simulink model "Hybrid_P2_Parallel"  (R2017b)
settings: Solver=FixedStepAuto  StartTime=0.0  StopTime=length(Speed)  FixedStep=0.01  MaxStep=0.01  RelTol=1e-3  EnableMultiTasking=on
PostLoadFcn:
  | , if any(exist('dsrtsu_mdlpostloadfcn', 'file') == [2, 3, 6]), try dsrtsu_mdlpostloadfcn('Execute', bdroot); catch fprintf('Error in PostLoadFcn (dsrtsu_mdlpostloadfcn) for model "%s":\n %s\n', bdroot, lasterr); end, end,
undefined symbols (not defined in the file): APP1_OOR, APP2_OOR, APP_Mismatch, Brk_Flt, cal, clt, Clutch, Clutch2, ClutchEngag, eng, Engine, EngOverTemp, ENGTRQ_MSMCH_Degraded_CP, ENGTRQ_MSMCH_ErrCritical_CP, ENGTRQ_MSMCH_LimpHome_CP, EngTrqMismatch, ess, ESSOverTemp, gb, KeyPos_Flt, LossCAN, MCUOverTemp, mot, MotDirMismatch, MotOverTemp, MotTrqMismatch, mph2kph, PRNDL_Flt, RegenFault, time, tloop
libraries: simulink x100, EC2_libraries x7, powerlib_meascontrol x2, lib_Actuators x1, CalculationGallon x1, lib_Chassis x1, autolibcoupling x1, autolibsharedcoupling x1, lib_DCDC x1, lib_Differential x1, lib_EMachine_2017a x1, lib_HVESS x1
(part 5 of 7)

== system Hybrid_P2_Parallel/Controller/HSC/Camaro Fault Detection/Input Conversions/BMS_Conversions/Override  closeContactorsCmd ==
  note: Override Switch Subsystem
  note: This subsystem is used to override the model value of a signal to a constant value
  In1 : Inport
  Multiport Switch : MultiPortSwitch  DataPortOrder=Zero-based contiguous  Inputs=2  zeroidx=on
  Override Value : Constant  Value=0  OutDataTypeStr=double
  Signal Override Switch 0 = Use Model 1 = Use Constant : Constant  Value=0
  Out1 : Outport
  wires:
  Override Value/1 -> Multiport Switch/3
  Multiport Switch/1 -> Out1/1
  In1/1 -> Multiport Switch/2
  Signal Override Switch 0 = Use Model 1 = Use Constant/1 -> Multiport Switch/1

== system Hybrid_P2_Parallel/Controller/HSC/Camaro Fault Detection/Input Conversions/BMS_Conversions/Override  contactorsClsd ==
  note: Override Switch Subsystem
  note: This subsystem is used to override the model value of a signal to a constant value
  In1 : Inport
  Multiport Switch : MultiPortSwitch  DataPortOrder=Zero-based contiguous  Inputs=2  zeroidx=on
  Override Value : Constant  Value=0  OutDataTypeStr=double
  Signal Override Switch 0 = Use Model 1 = Use Constant : Constant  Value=0
  Out1 : Outport
  wires:
  Override Value/1 -> Multiport Switch/3
  Multiport Switch/1 -> Out1/1
  In1/1 -> Multiport Switch/2
  Signal Override Switch 0 = Use Model 1 = Use Constant/1 -> Multiport Switch/1

== system Hybrid_P2_Parallel/Controller/HSC/Camaro Fault Detection/Input Conversions/BMS_Conversions/Override  essCur_A ==
  note: This subsystem is used to override the model value of a signal to a constant value
  note: Override Switch Subsystem
  In1 : Inport
  Multiport Switch : MultiPortSwitch  DataPortOrder=Zero-based contiguous  Inputs=2  zeroidx=on
  Override Value : Constant  Value=0  OutDataTypeStr=double
  Signal Override Switch 0 = Use Model 1 = Use Constant : Constant  Value=0
  Out1 : Outport
  wires:
  Signal Override Switch 0 = Use Model 1 = Use Constant/1 -> Multiport Switch/1
  In1/1 -> Multiport Switch/2
  Multiport Switch/1 -> Out1/1
  Override Value/1 -> Multiport Switch/3

== system Hybrid_P2_Parallel/Controller/HSC/Camaro Fault Detection/Input Conversions/BMS_Conversions/Override  essSOC_0_1 ==
  note: Override Switch Subsystem
  note: This subsystem is used to override the model value of a signal to a constant value
  In1 : Inport
  Multiport Switch : MultiPortSwitch  DataPortOrder=Zero-based contiguous  Inputs=2  zeroidx=on
  Override Value : Constant  Value=0  OutDataTypeStr=double
  Signal Override Switch 0 = Use Model 1 = Use Constant : Constant  Value=0
  Out1 : Outport
  wires:
  Override Value/1 -> Multiport Switch/3
  Multiport Switch/1 -> Out1/1
  In1/1 -> Multiport Switch/2
  Signal Override Switch 0 = Use Model 1 = Use Constant/1 -> Multiport Switch/1

== system Hybrid_P2_Parallel/Controller/HSC/Camaro Fault Detection/Input Conversions/BMS_Conversions/Override  essTemp_C ==
  note: Override Switch Subsystem
  note: This subsystem is used to override the model value of a signal to a constant value
  In1 : Inport
  Multiport Switch : MultiPortSwitch  DataPortOrder=Zero-based contiguous  Inputs=2  zeroidx=on
  Override Value : Constant  Value=0  OutDataTypeStr=double
  Signal Override Switch 0 = Use Model 1 = Use Constant : Constant
  Out1 : Outport
  wires:
  Override Value/1 -> Multiport Switch/3
  Multiport Switch/1 -> Out1/1
  In1/1 -> Multiport Switch/2
  Signal Override Switch 0 = Use Model 1 = Use Constant/1 -> Multiport Switch/1

== system Hybrid_P2_Parallel/Controller/HSC/Camaro Fault Detection/Input Conversions/BMS_Conversions/Override  hvBattVolt_V ==
  note: Override Switch Subsystem
  note: This subsystem is used to override the model value of a signal to a constant value
  In1 : Inport
  Multiport Switch : MultiPortSwitch  DataPortOrder=Zero-based contiguous  Inputs=2  zeroidx=on
  Override Value : Constant  Value=0  OutDataTypeStr=double
  Signal Override Switch 0 = Use Model 1 = Use Constant : Constant  Value=0
  Out1 : Outport
  wires:
  Override Value/1 -> Multiport Switch/3
  Multiport Switch/1 -> Out1/1
  In1/1 -> Multiport Switch/2
  Signal Override Switch 0 = Use Model 1 = Use Constant/1 -> Multiport Switch/1

== system Hybrid_P2_Parallel/Controller/HSC/Camaro Fault Detection/Input Conversions/BMS_Conversions/Override  hvBusVolt_V ==
  note: This subsystem is used to override the model value of a signal to a constant value
  note: Override Switch Subsystem
  In1 : Inport
  Multiport Switch : MultiPortSwitch  DataPortOrder=Zero-based contiguous  Inputs=2  zeroidx=on
  Override Value : Constant  Value=0  OutDataTypeStr=double
  Signal Override Switch 0 = Use Model 1 = Use Constant : Constant  Value=0
  Out1 : Outport
  wires:
  Signal Override Switch 0 = Use Model 1 = Use Constant/1 -> Multiport Switch/1
  In1/1 -> Multiport Switch/2
  Multiport Switch/1 -> Out1/1
  Override Value/1 -> Multiport Switch/3

== system Hybrid_P2_Parallel/Controller/HSC/Camaro Fault Detection/Input Conversions/BMS_Conversions/Override  rollingAliveCnt [1_3] ==
  note: This subsystem is used to override the model value of a signal to a constant value
  note: Override Switch Subsystem
  In1 : Inport
  Multiport Switch : MultiPortSwitch  DataPortOrder=Zero-based contiguous  Inputs=2  zeroidx=on
  Override Value : Constant  Value=0  OutDataTypeStr=double
  Signal Override Switch 0 = Use Model 1 = Use Constant : Constant  Value=0
  Out1 : Outport
  wires:
  Signal Override Switch 0 = Use Model 1 = Use Constant/1 -> Multiport Switch/1
  In1/1 -> Multiport Switch/2
  Multiport Switch/1 -> Out1/1
  Override Value/1 -> Multiport Switch/3

== system Hybrid_P2_Parallel/Controller/HSC/Camaro Fault Detection/Input Conversions/BMS_Conversions/Override Fehler_HS_offen ==
  note: Override Switch Subsystem
  note: This subsystem is used to override the model value of a signal to a constant value
  In1 : Inport
  Multiport Switch : MultiPortSwitch  DataPortOrder=Zero-based contiguous  Inputs=2  zeroidx=on
  Override Value : Constant  Value=0  OutDataTypeStr=double
  Signal Override Switch 0 = Use Model 1 = Use Constant : Constant
  Out1 : Outport
  wires:
  Override Value/1 -> Multiport Switch/3
  Multiport Switch/1 -> Out1/1
  In1/1 -> Multiport Switch/2
  Signal Override Switch 0 = Use Model 1 = Use Constant/1 -> Multiport Switch/1

== system Hybrid_P2_Parallel/Controller/HSC/Camaro Fault Detection/Input Conversions/BMS_Conversions/Override Fehler_HS_verschweisst ==
  note: This subsystem is used to override the model value of a signal to a constant value
  note: Override Switch Subsystem
  In1 : Inport
  Multiport Switch : MultiPortSwitch  DataPortOrder=Zero-based contiguous  Inputs=2  zeroidx=on
  Override Value : Constant  Value=0  OutDataTypeStr=double
  Signal Override Switch 0 = Use Model 1 = Use Constant : Constant
  Out1 : Outport
  wires:
  Signal Override Switch 0 = Use Model 1 = Use Constant/1 -> Multiport Switch/1
  In1/1 -> Multiport Switch/2
  Multiport Switch/1 -> Out1/1
  Override Value/1 -> Multiport Switch/3

== system Hybrid_P2_Parallel/Controller/HSC/Camaro Fault Detection/Input Conversions/DriverInput_Conversions/Override  KeyPos [0_3] ==
  note: This subsystem is used to override the model value of a signal to a constant value
  note: Override Switch Subsystem
  In1 : Inport
  Multiport Switch : MultiPortSwitch  DataPortOrder=Zero-based contiguous  Inputs=2  zeroidx=on
  Override Value : Constant  Value=0  OutDataTypeStr=double
  Signal Override Switch 0 = Use Model 1 = Use Constant : Constant  Value=0
  Out1 : Outport
  wires:
  Signal Override Switch 0 = Use Model 1 = Use Constant/1 -> Multiport Switch/1
  In1/1 -> Multiport Switch/2
  Multiport Switch/1 -> Out1/1
  Override Value/1 -> Multiport Switch/3

== system Hybrid_P2_Parallel/Controller/HSC/Camaro Fault Detection/Input Conversions/DriverInput_Conversions/Override APP (%) ==
  note: This subsystem is used to override the model value of a signal to a constant value
  note: Override Switch Subsystem
  In1 : Inport
  Multiport Switch : MultiPortSwitch  DataPortOrder=Zero-based contiguous  Inputs=2  zeroidx=on
  Override Value : Constant  Value=0  OutDataTypeStr=double
  Signal Override Switch 0 = Use Model 1 = Use Constant : Constant  Value=0
  Out1 : Outport
  wires:
  Signal Override Switch 0 = Use Model 1 = Use Constant/1 -> Multiport Switch/1
  In1/1 -> Multiport Switch/2
  Multiport Switch/1 -> Out1/1
  Override Value/1 -> Multiport Switch/3

== system Hybrid_P2_Parallel/Controller/HSC/Camaro Fault Detection/Input Conversions/DriverInput_Conversions/Override APP (%)1 ==
  note: Override Switch Subsystem
  note: This subsystem is used to override the model value of a signal to a constant value
  In1 : Inport
  Multiport Switch : MultiPortSwitch  DataPortOrder=Zero-based contiguous  Inputs=2  zeroidx=on
  Override Value : Constant  Value=0  OutDataTypeStr=double
  Signal Override Switch 0 = Use Model 1 = Use Constant : Constant  Value=0
  Out1 : Outport
  wires:
  Override Value/1 -> Multiport Switch/3
  Multiport Switch/1 -> Out1/1
  In1/1 -> Multiport Switch/2
  Signal Override Switch 0 = Use Model 1 = Use Constant/1 -> Multiport Switch/1

== system Hybrid_P2_Parallel/Controller/HSC/Camaro Fault Detection/Input Conversions/DriverInput_Conversions/Override BPP (%) ==
  note: Override Switch Subsystem
  note: This subsystem is used to override the model value of a signal to a constant value
  In1 : Inport
  Multiport Switch : MultiPortSwitch  DataPortOrder=Zero-based contiguous  Inputs=2  zeroidx=on
  Override Value : Constant  Value=0  OutDataTypeStr=double
  Signal Override Switch 0 = Use Model 1 = Use Constant : Constant  Value=0
  Out1 : Outport
  wires:
  Override Value/1 -> Multiport Switch/3
  Multiport Switch/1 -> Out1/1
  In1/1 -> Multiport Switch/2
  Signal Override Switch 0 = Use Model 1 = Use Constant/1 -> Multiport Switch/1

== system Hybrid_P2_Parallel/Controller/HSC/Camaro Fault Detection/Input Conversions/DriverInput_Conversions/Override PRNDL ==
  note: This subsystem is used to override the model value of a signal to a constant value
  note: Override Switch Subsystem
  In1 : Inport
  Multiport Switch : MultiPortSwitch  DataPortOrder=Zero-based contiguous  Inputs=2  zeroidx=on
  Override Value : Constant  Value=0  OutDataTypeStr=double
  Signal Override Switch 0 = Use Model 1 = Use Constant : Constant  Value=0
  Out1 : Outport
  wires:
  Signal Override Switch 0 = Use Model 1 = Use Constant/1 -> Multiport Switch/1
  In1/1 -> Multiport Switch/2
  Multiport Switch/1 -> Out1/1
  Override Value/1 -> Multiport Switch/3

== system Hybrid_P2_Parallel/Controller/HSC/Camaro Fault Detection/Input Conversions/DriverInput_Conversions/Override Regen ==
  note: This subsystem is used to override the model value of a signal to a constant value
  note: Override Switch Subsystem
  In1 : Inport
  Multiport Switch : MultiPortSwitch  DataPortOrder=Zero-based contiguous  Inputs=2  zeroidx=on
  Override Value : Constant  Value=0  OutDataTypeStr=double
  Signal Override Switch 0 = Use Model 1 = Use Constant : Constant  Value=0
  Out1 : Outport
  wires:
  Signal Override Switch 0 = Use Model 1 = Use Constant/1 -> Multiport Switch/1
  In1/1 -> Multiport Switch/2
  Multiport Switch/1 -> Out1/1
  Override Value/1 -> Multiport Switch/3

== system Hybrid_P2_Parallel/Controller/HSC/Camaro Fault Detection/Input Conversions/DriverInput_Conversions/Override V [mph] ==
  note: Override Switch Subsystem
  note: This subsystem is used to override the model value of a signal to a constant value
  In1 : Inport
  Multiport Switch : MultiPortSwitch  DataPortOrder=Zero-based contiguous  Inputs=2  zeroidx=on
  Override Value : Constant  Value=0  OutDataTypeStr=double
  Signal Override Switch 0 = Use Model 1 = Use Constant : Constant  Value=0
  Out1 : Outport
  wires:
  Override Value/1 -> Multiport Switch/3
  Multiport Switch/1 -> Out1/1
  In1/1 -> Multiport Switch/2
  Signal Override Switch 0 = Use Model 1 = Use Constant/1 -> Multiport Switch/1

== system Hybrid_P2_Parallel/Controller/HSC/Camaro Fault Detection/Input Conversions/ECM_Conversions/Override  ECMTrqCmd_Nm ==
  note: Override Switch Subsystem
  note: This subsystem is used to override the model value of a signal to a constant value
  In1 : Inport
  Multiport Switch : MultiPortSwitch  DataPortOrder=Zero-based contiguous  Inputs=2  zeroidx=on
  Override Value : Constant  Value=0  OutDataTypeStr=double
  Signal Override Switch 0 = Use Model 1 = Use Constant : Constant  Value=0
  Out1 : Outport
  wires:
  Override Value/1 -> Multiport Switch/3
  Multiport Switch/1 -> Out1/1
  In1/1 -> Multiport Switch/2
  Signal Override Switch 0 = Use Model 1 = Use Constant/1 -> Multiport Switch/1

== system Hybrid_P2_Parallel/Controller/HSC/Camaro Fault Detection/Input Conversions/ECM_Conversions/Override  ECMrollingAliveCnt ==
  note: This subsystem is used to override the model value of a signal to a constant value
  note: Override Switch Subsystem
  In1 : Inport
  Multiport Switch : MultiPortSwitch  DataPortOrder=Zero-based contiguous  Inputs=2  zeroidx=on
  Override Value : Constant  Value=0  OutDataTypeStr=double
  Signal Override Switch 0 = Use Model 1 = Use Constant : Constant  Value=0
  Out1 : Outport
  wires:
  Signal Override Switch 0 = Use Model 1 = Use Constant/1 -> Multiport Switch/1
  In1/1 -> Multiport Switch/2
  Multiport Switch/1 -> Out1/1
  Override Value/1 -> Multiport Switch/3

== system Hybrid_P2_Parallel/Controller/HSC/Camaro Fault Detection/Input Conversions/ECM_Conversions/Override  EngActStdyStTorq_Nm ==
  note: This subsystem is used to override the model value of a signal to a constant value
  note: Override Switch Subsystem
  In1 : Inport
  Multiport Switch : MultiPortSwitch  DataPortOrder=Zero-based contiguous  Inputs=2  zeroidx=on
  Override Value : Constant  Value=0  OutDataTypeStr=double
  Signal Override Switch 0 = Use Model 1 = Use Constant : Constant  Value=0
  Out1 : Outport
  wires:
  Signal Override Switch 0 = Use Model 1 = Use Constant/1 -> Multiport Switch/1
  In1/1 -> Multiport Switch/2
  Multiport Switch/1 -> Out1/1
  Override Value/1 -> Multiport Switch/3

== system Hybrid_P2_Parallel/Controller/HSC/Camaro Fault Detection/Input Conversions/ECM_Conversions/Override  EngRunAtv ==
  note: Override Switch Subsystem
  note: This subsystem is used to override the model value of a signal to a constant value
  In1 : Inport
  Multiport Switch : MultiPortSwitch  DataPortOrder=Zero-based contiguous  Inputs=2  zeroidx=on
  Override Value : Constant  Value=0  OutDataTypeStr=double
  Signal Override Switch 0 = Use Model 1 = Use Constant : Constant  Value=0
  Out1 : Outport
  wires:
  Override Value/1 -> Multiport Switch/3
  Multiport Switch/1 -> Out1/1
  In1/1 -> Multiport Switch/2
  Signal Override Switch 0 = Use Model 1 = Use Constant/1 -> Multiport Switch/1

== system Hybrid_P2_Parallel/Controller/HSC/Camaro Fault Detection/Input Conversions/ECM_Conversions/Override  EngineSpeed_rpm ==
  note: Override Switch Subsystem
  note: This subsystem is used to override the model value of a signal to a constant value
  In1 : Inport
  Multiport Switch : MultiPortSwitch  DataPortOrder=Zero-based contiguous  Inputs=2  zeroidx=on
  Override Value : Constant  Value=0  OutDataTypeStr=double
  Signal Override Switch 0 = Use Model 1 = Use Constant : Constant  Value=0
  Out1 : Outport
  wires:
  Override Value/1 -> Multiport Switch/3
  Multiport Switch/1 -> Out1/1
  In1/1 -> Multiport Switch/2
  Signal Override Switch 0 = Use Model 1 = Use Constant/1 -> Multiport Switch/1

== system Hybrid_P2_Parallel/Controller/HSC/Camaro Fault Detection/Input Conversions/ECM_Conversions/Override  Engine_Temp[DegC] ==
  note: This subsystem is used to override the model value of a signal to a constant value
  note: Override Switch Subsystem
  In1 : Inport
  Multiport Switch : MultiPortSwitch  DataPortOrder=Zero-based contiguous  Inputs=2  zeroidx=on
  Override Value : Constant  Value=0  OutDataTypeStr=double
  Signal Override Switch 0 = Use Model 1 = Use Constant : Constant  Value=0
  Out1 : Outport
  wires:
  Signal Override Switch 0 = Use Model 1 = Use Constant/1 -> Multiport Switch/1
  In1/1 -> Multiport Switch/2
  Multiport Switch/1 -> Out1/1
  Override Value/1 -> Multiport Switch/3

== system Hybrid_P2_Parallel/Controller/HSC/Camaro Fault Detection/Input Conversions/TCM_Conversions/Override  LockupCmd ==
  note: Override Switch Subsystem
  note: This subsystem is used to override the model value of a signal to a constant value
  In1 : Inport
  Multiport Switch : MultiPortSwitch  DataPortOrder=Zero-based contiguous  Inputs=2  zeroidx=on
  Override Value : Constant  Value=0  OutDataTypeStr=double
  Signal Override Switch 0 = Use Model 1 = Use Constant : Constant  Value=0
  Out1 : Outport
  wires:
  Override Value/1 -> Multiport Switch/3
  Multiport Switch/1 -> Out1/1
  In1/1 -> Multiport Switch/2
  Signal Override Switch 0 = Use Model 1 = Use Constant/1 -> Multiport Switch/1

== system Hybrid_P2_Parallel/Controller/HSC/Camaro Fault Detection/Input Conversions/TCM_Conversions/Override  LvrPosTrnsShft  ==
  note: Override Switch Subsystem
  note: This subsystem is used to override the model value of a signal to a constant value
  In1 : Inport
  Multiport Switch : MultiPortSwitch  DataPortOrder=Zero-based contiguous  Inputs=2  zeroidx=on
  Override Value : Constant  Value=0  OutDataTypeStr=double
  Signal Override Switch 0 = Use Model 1 = Use Constant : Constant  Value=0
  Out1 : Outport
  wires:
  Override Value/1 -> Multiport Switch/3
  Multiport Switch/1 -> Out1/1
  In1/1 -> Multiport Switch/2
  Signal Override Switch 0 = Use Model 1 = Use Constant/1 -> Multiport Switch/1

== system Hybrid_P2_Parallel/Controller/HSC/Camaro Fault Detection/Input Conversions/TCM_Conversions/Override  TransEstGear ==
  note: Override Switch Subsystem
  note: This subsystem is used to override the model value of a signal to a constant value
  In1 : Inport
  Multiport Switch : MultiPortSwitch  DataPortOrder=Zero-based contiguous  Inputs=2  zeroidx=on
  Override Value : Constant  Value=0  OutDataTypeStr=double
  Signal Override Switch 0 = Use Model 1 = Use Constant : Constant  Value=0
  Out1 : Outport
  wires:
  Override Value/1 -> Multiport Switch/3
  Multiport Switch/1 -> Out1/1
  In1/1 -> Multiport Switch/2
  Signal Override Switch 0 = Use Model 1 = Use Constant/1 -> Multiport Switch/1

== system Hybrid_P2_Parallel/Controller/HSC/Camaro Fault Detection/Input Conversions/TCM_Conversions/Override  rollingAliveCnt [123] ==
  note: Override Switch Subsystem
  note: This subsystem is used to override the model value of a signal to a constant value
  In1 : Inport
  Multiport Switch : MultiPortSwitch  DataPortOrder=Zero-based contiguous  Inputs=2  zeroidx=on
  Override Value : Constant  Value=0  OutDataTypeStr=double
  Signal Override Switch 0 = Use Model 1 = Use Constant : Constant  Value=0
  Out1 : Outport
  wires:
  Override Value/1 -> Multiport Switch/3
  Multiport Switch/1 -> Out1/1
  In1/1 -> Multiport Switch/2
  Signal Override Switch 0 = Use Model 1 = Use Constant/1 -> Multiport Switch/1

== system Hybrid_P2_Parallel/Controller/HSC/Camaro Fault Detection/Input Conversions/TCM_Conversions/TCM_RollinAliveCounter ==
  Constant : Constant  Value=0
  Constant8 : Constant
  Rolling Alive Counter1 : Stateflow chart  TreatAsAtomicUnit=on
  Switch1 : Switch  Criteria=u2 > Threshold
  Out1 : Outport
  wires:
  Constant8/1 -> Switch1/1
  Rolling Alive Counter1/1(RollingAliveCnt) -> Switch1/3
  [TCM_CAN_fault] -> Switch1/2
  Switch1/1 -> Out1/1  "TCMRollingAliveCnt [0 1 2 3]"
  Constant/1 -> [TCM_CAN_fault]

== system Hybrid_P2_Parallel/Controller/HSC/Camaro Fault Detection/Signal Diagnostic/Driver Signal Diagnostic/APP_Crosscheck ==
  In1 : Inport
  In2 : Inport  Port=2
  Abs : Abs
  Compare To Constant : simulink/Logic and Bit Operations/Compare To Constant  relop=<=  const=0.5  OutDataTypeStr=boolean
  Sum : Sum  Inputs=+-
  Out1 : Outport
  wires:
  Compare To Constant/1 -> Out1/1  "Drv_APP_Agree"
  In2/1 -> Sum/2
  In1/1 -> Sum/1
  Abs/1 -> Compare To Constant/1
  Sum/1 -> Abs/1

== system Hybrid_P2_Parallel/Controller/HSC/Camaro Fault Detection/Signal Diagnostic/Driver Signal Diagnostic/BrakeFailureDetection ==
  BPP : Inport
  VehSpeed : Inport  Port=2
  Trigger : TriggerPort  VariantControl=Variant  PortDimensions=1
  Chart : Stateflow chart  Commented=on  TreatAsAtomicUnit=on
  Compare To Constant : simulink/Logic and Bit Operations/Compare To Constant  relop=>  const=0  OutDataTypeStr=boolean
  Compare To Constant1 : simulink/Logic and Bit Operations/Compare To Constant  relop=>  const=0.5  OutDataTypeStr=boolean
  Detect Change : simulink/Logic and Bit Operations/Detect Change  vinit=0  InputProcessing=Inherited  OutDataTypeStr=boolean
  Detect Increase : simulink/Logic and Bit Operations/Detect Increase  vinit=0.0  InputProcessing=Inherited  OutDataTypeStr=boolean
  Logical Operator : Logic  Operator=NOT  AllPortsSameDT=off  OutDataTypeStr=boolean
  Logical Operator1 : Logic  AllPortsSameDT=off  OutDataTypeStr=boolean
  Logical Operator2 : Logic  Operator=OR  AllPortsSameDT=off  OutDataTypeStr=boolean
  Logical Operator3 : Logic  AllPortsSameDT=off  OutDataTypeStr=boolean
  Unit Delay : UnitDelay  SampleTime=-1
  Unit Delay1 : UnitDelay  SampleTime=-1
  DecelFail : Outport
  wires:
  Logical Operator3/1 -> DecelFail/1
  Logical Operator2/1 -> Logical Operator3/2
  Unit Delay1/1 -> Compare To Constant1/1
  Unit Delay/1 -> Compare To Constant/1
  Logical Operator/1 -> Logical Operator2/2  "Unchange"
  Detect Increase/1 -> Logical Operator2/1  "Increase"
  Logical Operator1/1 -> Logical Operator3/1
  BPP/1 -> Unit Delay/1
  Compare To Constant1/1 -> Logical Operator1/2
  Compare To Constant/1 -> Logical Operator1/1
  Detect Change/1 -> Logical Operator/1
  VehSpeed/1 -> Detect Increase/1, Detect Change/1, Unit Delay1/1

== system Hybrid_P2_Parallel/Controller/HSC/Camaro Fault Detection/Signal Diagnostic/Driver Signal Diagnostic/Latch ==
  In1 : Inport
  In2 : Inport  Port=2
  Memory : Memory
  NOT : Logic  Operator=NOT  OutDataTypeStr=boolean
  OR : Logic  OutDataTypeStr=boolean
  OR1 : Logic  Operator=OR  OutDataTypeStr=boolean
  Drv_APP_Agree : Outport
  wires:
  In2/1 -> NOT/1
  Memory/1 -> OR/2
  NOT/1 -> OR/1
  OR1/1 -> Memory/1, Drv_APP_Agree/1
  OR/1 -> OR1/2
  In1/1 -> OR1/1

== system Hybrid_P2_Parallel/Controller/HSC/Camaro Fault Detection/Signal Diagnostic/Driver Signal Diagnostic/Latch1 ==
  In1 : Inport
  In2 : Inport  Port=2
  Memory : Memory
  NOT : Logic  Operator=NOT  OutDataTypeStr=boolean
  OR : Logic  OutDataTypeStr=boolean
  OR1 : Logic  Operator=OR  OutDataTypeStr=boolean
  Out1 : Outport
  wires:
  In1/1 -> OR1/1
  OR/1 -> OR1/2
  OR1/1 -> Out1/1, Memory/1
  NOT/1 -> OR/1
  Memory/1 -> OR/2
  In2/1 -> NOT/1

== system Hybrid_P2_Parallel/Controller/HSC/Camaro Fault Detection/Signal Diagnostic/ESS Signal Diagnostic/Contactors status check ==
  note: Note: Contactors don't close when commanded
  In1 : Inport
  In2 : Inport  Port=2
  In3 : Inport  Port=3
  " " : simulink/Logic and Bit Operations/Compare To Constant  relop=>  const=0.5  OutDataTypeStr=boolean
  Abs : Abs
  Logical Operator : Logic  Operator=OR  AllPortsSameDT=off  OutDataTypeStr=boolean
  Sum : Sum  Inputs=+-
  Out1 : Outport
  wires:
  In1/1 -> Sum/1
  Logical Operator/1 -> Out1/1  "BMS_contactorsFailed_Detected"
  Sum/1 -> Abs/1
  Abs/1 -> " "/1
  In2/1 -> Sum/2
  In3/1 -> Logical Operator/2
  " "/1 -> Logical Operator/1  "BMS_contactorsFailed_SigValid"

== system Hybrid_P2_Parallel/Controller/HSC/Camaro Fault Detection/Signal Diagnostic/ESS Signal Diagnostic/ESS SOC Validity Check ==
  In1 : Inport
  Constant1 : Constant
  essSOCValidity_Check : Subsystem
  essSOC_0_1Range : Stateflow chart  TreatAsAtomicUnit=on
  Out1 : Outport
  Out2 : Outport  Port=2
  wires:
  essSOC_0_1Range/1(essSOCRange) -> essSOCValidity_Check/1(In1), Out2/1
  Constant1/1 -> essSOC_0_1Range/1(clearFaults)
  In1/1 -> essSOC_0_1Range/2(signalValue)
  essSOCValidity_Check/1(Out1) -> Out1/1  "BMS_essSOC_0_1_SigValid"

== system Hybrid_P2_Parallel/Controller/HSC/Camaro Fault Detection/Signal Diagnostic/ESS Signal Diagnostic/ESS Temp Validity Check ==
  In1 : Inport
  Constant : Constant
  essTsignalRange : Stateflow chart  TreatAsAtomicUnit=on
  essTsignalValidity_Check : Subsystem
  Out1 : Outport
  Out2 : Outport  Port=2
  wires:
  In1/1 -> essTsignalRange/2(signalValue)
  essTsignalRange/1(essTempRange) -> essTsignalValidity_Check/1(In1), Out2/1  "essTempRange[0_4]"
  essTsignalValidity_Check/1(Out1) -> Out1/1  "BMS_essTemp_[degC]_SigValid"
  Constant/1 -> essTsignalRange/1(clearFaults)

== system Hybrid_P2_Parallel/Controller/HSC/Camaro Fault Detection/Signal Diagnostic/ESS Signal Diagnostic/Max charging voltage fault detect ==
  note: Note: When the ESS receives the energy from grid or regenerative braking,
      | the charging voltage to the inverter can not be bigger than 419V, otherwise the MCU will set to fault
  In1 : Inport
  " " : simulink/Logic and Bit Operations/Compare To Constant  relop=>  const=419  OutDataTypeStr=boolean
  Abs : Abs
  Compare To Zero : simulink/Logic and Bit Operations/Compare To Zero  relop=<  OutDataTypeStr=boolean
  Logical Operator : Logic  AllPortsSameDT=off  OutDataTypeStr=boolean
  Out1 : Outport
  wires:
  Abs/1 -> " "/1
  Logical Operator/1 -> Out1/1
  " "/1 -> Logical Operator/1
  In1/1 -> Compare To Zero/1, Abs/1
  Compare To Zero/1 -> Logical Operator/2

== system Hybrid_P2_Parallel/Controller/HSC/Camaro Fault Detection/Signal Diagnostic/ESS Signal Diagnostic/Rolling Alive Counter Detection ==
  In1 : Inport
  Chart : Stateflow chart  TreatAsAtomicUnit=on
  Constant : Constant  Value=0.01
  Constant1 : Constant  Value=0.01
  Detect Change : simulink/Logic and Bit Operations/Detect Change  vinit=1  InputProcessing=Inherited  OutDataTypeStr=boolean
  Out1 : Outport
  wires:
  Constant1/1 -> Chart/3(tloop)
  In1/1 -> Detect Change/1
  Detect Change/1 -> Chart/1(PulseDetect)
  Chart/1(flag) -> Out1/1
  Constant/1 -> Chart/2(CycleTime)

== system Hybrid_P2_Parallel/Controller/HSC/Camaro Fault Detection/Signal Diagnostic/ESS Signal Diagnostic/Validity Check ==
  In1 : Inport
  " Normal Operation" : simulink/Logic and Bit Operations/Compare To Constant  relop===  const=1  OutDataTypeStr=boolean
  Below Normal Operation : simulink/Logic and Bit Operations/Compare To Constant  relop===  const=0  OutDataTypeStr=boolean
  Logical Operator : Logic  Operator=OR  AllPortsSameDT=off  OutDataTypeStr=boolean
  Out1 : Outport
  wires:
  In1/1 -> Below Normal Operation/1, " Normal Operation"/1
  Below Normal Operation/1 -> Logical Operator/1
  " Normal Operation"/1 -> Logical Operator/2
  Logical Operator/1 -> Out1/1  "BMSgdf_SigValid"

== system Hybrid_P2_Parallel/Controller/HSC/Camaro Fault Detection/Signal Diagnostic/Engine Signal Diagnostic/EngTempValidity_Check ==
  In1 : Inport
  Above Normal Operation : simulink/Logic and Bit Operations/Compare To Constant  relop===  const=3  OutDataTypeStr=boolean
  Logical Operator1 : Logic  Operator=NOT  AllPortsSameDT=off  OutDataTypeStr=boolean
  Out1 : Outport
  wires:
  Logical Operator1/1 -> Out1/1
  Above Normal Operation/1 -> Logical Operator1/1
  In1/1 -> Above Normal Operation/1

== system Hybrid_P2_Parallel/Controller/HSC/Camaro Fault Detection/Signal Diagnostic/Engine Signal Diagnostic/Rolling Alive Counter Detection1 ==
  In1 : Inport
  Chart : Stateflow chart  TreatAsAtomicUnit=on
  Constant : Constant  Value=0.01
  Detect Change : simulink/Logic and Bit Operations/Detect Change  vinit=1  InputProcessing=Inherited  OutDataTypeStr=boolean
  Out1 : Outport
  wires:
  Constant/1 -> Chart/2(CycleTime)
  Chart/1(flag) -> Out1/1
  Detect Change/1 -> Chart/1(PulseDetect)
  In1/1 -> Detect Change/1

== system Hybrid_P2_Parallel/Controller/HSC/Camaro Fault Detection/Signal Diagnostic/Transmission Signal Diagnostic/Rolling Alive Counter Detection ==
  In1 : Inport
  Chart : Stateflow chart  TreatAsAtomicUnit=on
  Constant : Constant  Value=0.01
  Detect Change : simulink/Logic and Bit Operations/Detect Change  vinit=1  InputProcessing=Inherited  OutDataTypeStr=boolean
  Out1 : Outport
  wires:
  Constant/1 -> Chart/2(CycleTime)
  Chart/1(flag) -> Out1/1
  Detect Change/1 -> Chart/1(PulseDetect)
  In1/1 -> Detect Change/1

== system Hybrid_P2_Parallel/Controller/HSC/Camaro Fault Detection/Signal Diagnostic/Transmission Signal Diagnostic/Vehicle Direction Fault Detection ==
  LvrPosTrnsShft : Inport
  Speed : Inport  Port=2
  Compare To Constant : simulink/Logic and Bit Operations/Compare To Constant  relop===  const=4  OutDataTypeStr=boolean
  Compare To Constant1 : simulink/Logic and Bit Operations/Compare To Constant  relop=<  const=0  OutDataTypeStr=boolean
  Compare To Constant2 : simulink/Logic and Bit Operations/Compare To Constant  relop===  const=2  OutDataTypeStr=boolean
  Compare To Constant3 : simulink/Logic and Bit Operations/Compare To Constant  relop=>  const=0  OutDataTypeStr=boolean
  Logical Operator : Logic  AllPortsSameDT=off  OutDataTypeStr=boolean
  Logical Operator1 : Logic  AllPortsSameDT=off  OutDataTypeStr=boolean
  Logical Operator2 : Logic  Operator=OR  AllPortsSameDT=off  OutDataTypeStr=boolean
  Out1 : Outport
  wires:
  Logical Operator2/1 -> Out1/1
  Logical Operator/1 -> Logical Operator2/2
  Logical Operator1/1 -> Logical Operator2/1
  Compare To Constant3/1 -> Logical Operator1/2
  Compare To Constant2/1 -> Logical Operator1/1
  Compare To Constant/1 -> Logical Operator/1
  Compare To Constant1/1 -> Logical Operator/2
  Speed/1 -> Compare To Constant1/1, Compare To Constant3/1
  LvrPosTrnsShft/1 -> Compare To Constant/1, Compare To Constant2/1

== system Hybrid_P2_Parallel/Controller/HSC/Driver_Requests/APP_BPP to DrvIntndAxlTrq2/Post Driver Intnded Axle Torque/Brake Command ==
  APP : Inport
  BPP : Inport  Port=2
  VehicleSpeed : Inport  Port=3
  1-D Lookup Table : Lookup_n-D  NumberOfTableDimensions=1  BreakpointsForDimension1=cal.Regen.BrakeAxleTrq.idx1_BrkPdlPos  Table=cal.Regen.BrakeAxleTrq.map  InternalRulePriority=Speed  RndMeth=Simplest  InputSameDT=on
  Compare To Constant : simulink/Logic and Bit Operations/Compare To Constant  relop=>=  const=cal.Regen.EnableSpeed  OutDataTypeStr=boolean
  Compare To Constant4 : simulink/Logic and Bit Operations/Compare To Constant  relop=<=  const=cal.Regen.EnableAPP  OutDataTypeStr=boolean
  Compare To Constant5 : simulink/Logic and Bit Operations/Compare To Constant  relop=>=  const=cal.Regen.DisableAPP  OutDataTypeStr=boolean
  Constant5 : Constant  Value=0
  Latch : Subsystem
  RegenCal : Gain  Gain=1.3
  Switch : Switch  Criteria=u2 > Threshold  Threshold=1
  Terminator : Terminator
  BrkAxlTrq : Outport
  wires:
  VehicleSpeed/1 -> Compare To Constant/1
  1-D Lookup Table/1 -> RegenCal/1
  Switch/1 -> BrkAxlTrq/1
  APP/1 -> Compare To Constant5/1, Compare To Constant4/1
  BPP/1 -> 1-D Lookup Table/1
  Compare To Constant/1 -> Switch/2
  Constant5/1 -> Switch/3
  Compare To Constant5/1 -> Latch/2(Reset)
  Compare To Constant4/1 -> Latch/1(Input)
  Latch/1(Out1) -> Terminator/1
  RegenCal/1 -> Switch/1

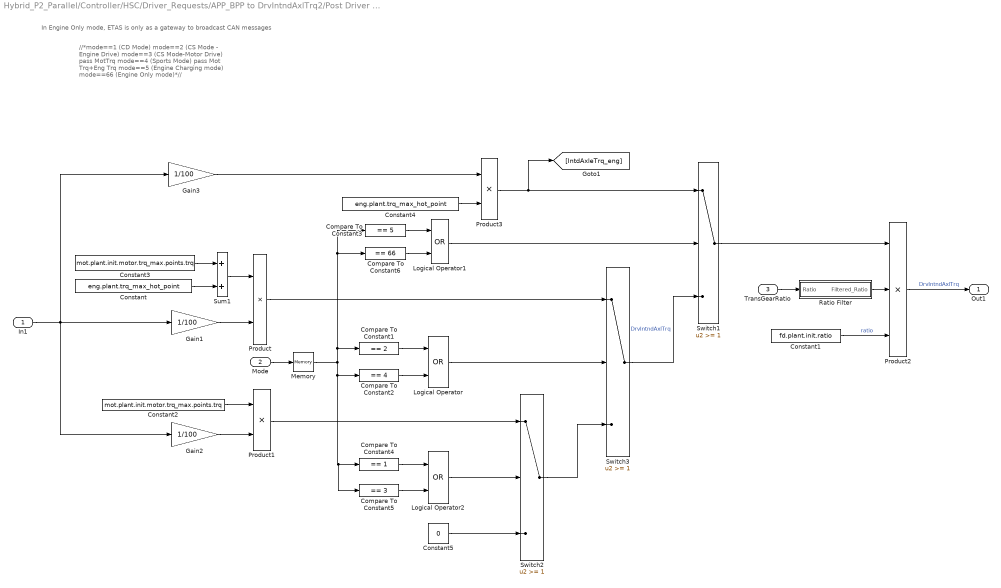
== system Hybrid_P2_Parallel/Controller/HSC/Driver_Requests/APP_BPP to DrvIntndAxlTrq2/Post Driver Intnded Axle Torque/Driver Intended Axle Torque ==
  note: In Engine Only mode, ETAS is only as a gateway to broadcast CAN messages
  note: //*mode==1 (CD Mode)
      | mode==2 (CS Mode - Engine Drive)
      | mode==3 (CS Mode-Motor Drive) pass MotTrq
      | mode==4 (Sports Mode) pass Mot Trq+Eng Trq
      | mode==5 (Engine Charging mode)
      | mode==66 (Engine Only mode)*//
  In1 : Inport
  Mode : Inport  Port=2
  TransGearRatio : Inport  Port=3
  Compare To Constant1 : simulink/Logic and Bit Operations/Compare To Constant  relop===  const=2  OutDataTypeStr=boolean
  Compare To Constant2 : simulink/Logic and Bit Operations/Compare To Constant  relop===  const=4  OutDataTypeStr=boolean
  Compare To Constant3 : simulink/Logic and Bit Operations/Compare To Constant  relop===  const=5  OutDataTypeStr=boolean
  Compare To Constant4 : simulink/Logic and Bit Operations/Compare To Constant  relop===  const=1  OutDataTypeStr=boolean
  Compare To Constant5 : simulink/Logic and Bit Operations/Compare To Constant  relop===  const=3  OutDataTypeStr=boolean
  Compare To Constant6 : simulink/Logic and Bit Operations/Compare To Constant  relop===  const=66  OutDataTypeStr=boolean
  Constant : Constant  Value=eng.plant.trq_max_hot_point  VectorParams1D=off
  Constant1 : Constant  Value=fd.plant.init.ratio
  Constant2 : Constant  Value=mot.plant.init.motor.trq_max.points.trq  VectorParams1D=off
  Constant3 : Constant  Value=mot.plant.init.motor.trq_max.points.trq  VectorParams1D=off
  Constant4 : Constant  Value=eng.plant.trq_max_hot_point  VectorParams1D=off
  Constant5 : Constant  Value=0
  Gain1 : Gain  Gain=1/100
  Gain2 : Gain  Gain=1/100
  Gain3 : Gain  Gain=1/100
  Logical Operator : Logic  Operator=OR  AllPortsSameDT=off  OutDataTypeStr=boolean
  Logical Operator1 : Logic  Operator=OR  AllPortsSameDT=off  OutDataTypeStr=boolean
  Logical Operator2 : Logic  Operator=OR  AllPortsSameDT=off  OutDataTypeStr=boolean
  Memory : Memory
  Product : Product  RndMeth=Zero
  Product1 : Product  RndMeth=Zero
  Product2 : Product  Inputs=3  RndMeth=Zero
  Product3 : Product  RndMeth=Zero
  Ratio Filter : Subsystem
  Sum1 : Sum
  Switch1 : Switch  Threshold=1
  Switch2 : Switch  Threshold=1
  Switch3 : Switch  Threshold=1
  Out1 : Outport
  wires:
  Constant2/1 -> Product1/1
  Ratio Filter/1(Filtered_Ratio) -> Product2/2
  Gain2/1 -> Product1/2
  Product/1 -> Switch3/1
  Mode/1 -> Memory/1
  Constant1/1 -> Product2/3  "ratio"
  Product1/1 -> Switch2/1
  TransGearRatio/1 -> Ratio Filter/1(Ratio)
  Product2/1 -> Out1/1  "DrvIntndAxlTrq"
  Gain1/1 -> Product/2
  Constant3/1 -> Sum1/1
  Compare To Constant1/1 -> Logical Operator/1
  Sum1/1 -> Product/1
  Compare To Constant2/1 -> Logical Operator/2
  Constant/1 -> Sum1/2
  Switch3/1 -> Switch1/3  "DrvIntndAxlTrq"
  Logical Operator/1 -> Switch3/2
  Product3/1 -> [IntdAxleTrq_eng], Switch1/1
  Switch1/1 -> Product2/1
  Compare To Constant3/1 -> Logical Operator1/1
  Memory/1 -> Compare To Constant3/1, Compare To Constant6/1, Compare To Constant1/1, Compare To Constant2/1, Compare To Constant5/1, Compare To Constant4/1
  In1/1 -> Gain2/1, Gain3/1, Gain1/1
  Constant4/1 -> Product3/2
  Gain3/1 -> Product3/1
  Logical Operator1/1 -> Switch1/2
  Compare To Constant6/1 -> Logical Operator1/2
  Switch2/1 -> Switch3/3
  Logical Operator2/1 -> Switch2/2
  Compare To Constant4/1 -> Logical Operator2/1
  Compare To Constant5/1 -> Logical Operator2/2
  Constant5/1 -> Switch2/3

== system Hybrid_P2_Parallel/Controller/HSC/Powertrain Manager/HV Manager/BMS_Manager/Fault Latch ==
  IsoFault : Inport
  Off Delay : powerlib_meascontrol/Logic/On Delay  DelayType=Off delay  delay=3  ic=0  Ts=0
      settings: SourceProductName=Simscape Power Systems
  IsoFaultLatched : Outport
  wires:
  IsoFault/1 -> Off Delay/1
  Off Delay/1 -> IsoFaultLatched/1

== system Hybrid_P2_Parallel/Controller/HSC/Powertrain Manager/HV Manager/BMS_Manager/ISO_Hybrid_01_Req ==
  In1 : Inport
  Bus Creator : BusCreator  Inputs=9
  ISO_Hybrid_01_Req_Data_byte_0 : Constant  Value=3
  ISO_Hybrid_01_Req_Data_byte_1 : Constant  Value=34
  ISO_Hybrid_01_Req_Data_byte_2 : Constant  Value=30
  ISO_Hybrid_01_Req_Data_byte_3 : Constant  Value=25
  ISO_Hybrid_01_Req_Data_byte_{4..7} (4 alike) : Constant  Value=0
  ISO_Hybrid_01_Req_Data_byte_8 : Constant  Value=23
  ISO_Request : DiscretePulseGenerator  PulseType=Time based  Period=0.5  PulseWidth=50  SampleTime=-1
  Switch{,1..8} (9 alike) : Switch  Criteria=u2 > Threshold
  Out1 : Outport
  wires:
  Bus Creator/1 -> Out1/1  "ISO_Hybrid_01_Req"
  Switch6/1 -> Bus Creator/6  "ISO_Hybrid_01_Req_Data_byte_5"
  ISO_Hybrid_01_Req_Data_byte_8/1 -> Switch/3
  Switch5/1 -> Bus Creator/5  "ISO_Hybrid_01_Req_Data_byte_4"
  Switch3/1 -> Bus Creator/3  "ISO_Hybrid_01_Req_Data_byte_2"
  ISO_Hybrid_01_Req_Data_byte_3/1 -> Switch/1
  Switch1/1 -> Bus Creator/1  "ISO_Hybrid_01_Req_Data_byte_0"
  Switch7/1 -> Bus Creator/7  "ISO_Hybrid_01_Req_Data_byte_6"
  Switch2/1 -> Bus Creator/2  "ISO_Hybrid_01_Req_Data_byte_1"
  Switch8/1 -> Bus Creator/8  "ISO_Hybrid_01_Req_Data_byte_7"
  Switch4/1 -> Bus Creator/4  "ISO_Hybrid_01_Req_Data_byte_3"
  ISO_Hybrid_01_Req_Data_byte_0/1 -> Switch1/1
  In1/1 -> Switch2/2, Switch3/3, Switch4/3, Switch5/3, Switch6/3, Switch7/2, Switch7/3, Switch8/2, Bus Creator/9, Switch8/3, Switch6/2, Switch5/2, Switch4/2, Switch3/2, Switch2/3, Switch1/3, Switch1/2
  ISO_Hybrid_01_Req_Data_byte_1/1 -> Switch2/1
  ISO_Hybrid_01_Req_Data_byte_2/1 -> Switch3/1
  Switch/1 -> Switch4/1  "ISO_Hybrid_01_Req_Data_byte_3"
  ISO_Hybrid_01_Req_Data_byte_4/1 -> Switch5/1
  ISO_Hybrid_01_Req_Data_byte_5/1 -> Switch6/1
  ISO_Hybrid_01_Req_Data_byte_6/1 -> Switch7/1
  ISO_Hybrid_01_Req_Data_byte_7/1 -> Switch8/1
  ISO_Request/1 -> Switch/2  "<ISO_Hybrid_01_Req_Data_byte_3>"

== system Hybrid_P2_Parallel/Controller/HSC/Powertrain Manager/HV Manager/BMS_Manager/Isolation Fault Calculation ==
  note: This block  allows to know which HV main
      | is having issues. HV POS 25, HV NEG 23.
  Sensors1 : Inport
  Bus Selector5 : BusSelector  OutputSignals=from_CAN.fromEBCAN.from_BMSAntrieb.ISO_Hybrid_01_Resp_Data.ISO_Hybrid_01_Resp_Data_byte_3,from_CAN.fromEBCAN.from_BMSAntrieb.ISO_Hybrid_01_Resp_Data.ISO_Hybrid_01_Resp_Data_byte_4,from_CAN.fromEBCAN.from_BMSAntrieb.ISO_Hybrid_01_Resp_Data.ISO_Hybrid_01_Resp_Data_byte_5
  Compare To Constant : simulink/Logic and Bit Operations/Compare To Constant  relop===  const=23  OutDataTypeStr=boolean
  Compare To Constant1 : simulink/Logic and Bit Operations/Compare To Constant  relop===  const=25  OutDataTypeStr=boolean
  HVnegativeISO : Constant  Value=0
  HVpositiveISO : Constant
  Logical Operator : Logic  Operator=OR  AllPortsSameDT=off  OutDataTypeStr=boolean
  POS or NEG HV MAIN : Switch  Criteria=u2 > Threshold  Threshold=24
  Resistance_Measurement : Subsystem
  Terminator8 : Terminator
  IsoFault : Outport
  wires:
  Resistance_Measurement/1(IsoFault) -> IsoFault/1
  POS or NEG HV MAIN/1 -> Terminator8/1
  Bus Selector5/2 -> Resistance_Measurement/1(In1)  "<ISO_Hybrid_01_Resp_Data_byte_4>"
  Bus Selector5/3 -> Resistance_Measurement/2(In2)  "<ISO_Hybrid_01_Resp_Data_byte_5>"
  Sensors1/1 -> Bus Selector5/1
  HVpositiveISO/1 -> POS or NEG HV MAIN/1
  Bus Selector5/1 -> POS or NEG HV MAIN/2, Compare To Constant1/1, Compare To Constant/1  "<ISO_Hybrid_01_Resp_Data_byte_3>"
  HVnegativeISO/1 -> POS or NEG HV MAIN/3
  Compare To Constant1/1 -> Logical Operator/1
  Compare To Constant/1 -> Logical Operator/2
  Logical Operator/1 -> Resistance_Measurement/Enable

== system Hybrid_P2_Parallel/Controller/HSC/Powertrain Manager/HV Manager/DCDC Manager/Contactors status check ==
  note: Note: Contactors don't close when commanded
  In1 : Inport
  " " : simulink/Logic and Bit Operations/Compare To Constant  relop=>  const=5  OutDataTypeStr=boolean
  Abs : Abs
  Bus Selector1 : BusSelector  OutputSignals=from_CAN.fromHV_CAN.from_BMSHybrid.BMS_HYB_02.BMS_IstSpannung,from_CAN.fromHV_CAN.from_BMSHybrid.BMS_Spannung_ZwKr,from_CAN.fromHV_CAN.from_BMSHybrid.BMS_HYB_02.BMS_Fehler_Pilot
  Logical Operator : Logic  Operator=OR  AllPortsSameDT=off  OutDataTypeStr=boolean
  Sum : Sum  Inputs=+-
  Out1 : Outport
  wires:
  Bus Selector1/1 -> Sum/1  "<BMS_IstSpannung>"
  Logical Operator/1 -> Out1/1  "BMS_contactorsFailed_Detected"
  Sum/1 -> Abs/1
  Abs/1 -> " "/1
  " "/1 -> Logical Operator/1  "BMS_contactorsFailed_SigValid"
  In1/1 -> Bus Selector1/1
  Bus Selector1/3 -> Logical Operator/2  "<BMS_Fehler_Pilot>"
  Bus Selector1/2 -> Sum/2  "<BMS_Spannung_ZwKr>"

== system Hybrid_P2_Parallel/Controller/HSC/Powertrain Manager/HV Manager/DCDC Manager/Subsystem ==
  In1 : Inport
  DCDCOVrrdSwitch : Constant  Value=0
  DCDCOVrrdVal : Constant  Value=0
  Switch : Switch  Criteria=u2 > Threshold
  Out1 : Outport
  wires:
  Switch/1 -> Out1/1  "DC_mode"
  In1/1 -> Switch/3
  DCDCOVrrdSwitch/1 -> Switch/2
  DCDCOVrrdVal/1 -> Switch/1

== system Hybrid_P2_Parallel/Controller/HSC/Powertrain Manager/HV Manager/DCDC Manager/Subsystem1 ==
  In1 : Inport
  Switch : Switch  Criteria=u2 > Threshold
  VoltageHVOvrrdSW : Constant  Value=0
  voltageHVOvrrdVal : Constant  Value=0
  Out1 : Outport
  wires:
  voltageHVOvrrdVal/1 -> Switch/1
  VoltageHVOvrrdSW/1 -> Switch/2
  In1/1 -> Switch/3
  Switch/1 -> Out1/1  "DC_mode"

== system Hybrid_P2_Parallel/Controller/HSC/Powertrain Manager/HV Manager/DCDC Manager/Subsystem2 ==
  In1 : Inport
  CurrentHVOvrrdSW : Constant  Value=0
  CurrentHVOvrrdVAL : Constant  Value=20
  Switch : Switch  Criteria=u2 > Threshold
  Out1 : Outport
  wires:
  Switch/1 -> Out1/1  "DC_mode"
  In1/1 -> Switch/3
  CurrentHVOvrrdSW/1 -> Switch/2
  CurrentHVOvrrdVAL/1 -> Switch/1

== system Hybrid_P2_Parallel/Controller/HSC/Powertrain Manager/HV Manager/DCDC Manager/Subsystem3 ==
  In1 : Inport
  Switch : Switch  Criteria=u2 > Threshold
  VoltageLVOvrrdSW : Constant  Value=0
  VoltageLVOvrrdVAL : Constant  Value=14
  Out1 : Outport
  wires:
  VoltageLVOvrrdVAL/1 -> Switch/1
  VoltageLVOvrrdSW/1 -> Switch/2
  In1/1 -> Switch/3
  Switch/1 -> Out1/1  "DC_mode"

== system Hybrid_P2_Parallel/Controller/HSC/Powertrain Manager/HV Manager/DCDC Manager/Subsystem4 ==
  In1 : Inport
  CurrentLVOvrrdSW : Constant  Value=0
  CurrentLVOvrrdVAL : Constant  Value=173
  Switch : Switch  Criteria=u2 > Threshold
  Out1 : Outport
  wires:
  Switch/1 -> Out1/1  "DC_mode"
  In1/1 -> Switch/3
  CurrentLVOvrrdSW/1 -> Switch/2
  CurrentLVOvrrdVAL/1 -> Switch/1

== system Hybrid_P2_Parallel/Controller/HSC/Powertrain Manager/Torque Distribution/AxlTrq_to_EngTrq/Ratio Filter ==
  Ratio : Inport
  Abs : Abs
  Compare To Zero : simulink/Logic and Bit Operations/Compare To Zero  relop===  OutDataTypeStr=boolean
  Constant : Constant  Value=cal.Time.TrnsOvrllEstTrqRatioSwitch
  Mature_Delay : EC2_libraries/Mature_Delay
  Memory1 : Memory  InitialCondition=1
  Switch1 : Switch  Threshold=1
  Switch2 : Switch  Threshold=1
  Filtered_Ratio : Outport
  wires:
  Switch2/1 -> Memory1/1, Filtered_Ratio/1  "gear_ratio"
  Memory1/1 -> Switch1/3
  Mature_Delay/1 -> Switch1/2
  Constant/1 -> Mature_Delay/2
  Switch1/1 -> Switch2/1
  Abs/1 -> Switch2/3, Switch1/1
  Compare To Zero/1 -> Switch2/2, Mature_Delay/1
  Ratio/1 -> Abs/1, Compare To Zero/1

== system Hybrid_P2_Parallel/Controller/HSC/Powertrain Manager/Torque Distribution/IdleMotTrq/AxlTrq_to_MotTrq ==
  In1 : Inport
  Mode : Inport  Port=2
  AxlTrq_to_MtrTrq2 : Subsystem
  MotTrqLimit : Saturate  UpperLimit=350  LowerLimit=-200
  RegTrqLimit : Subsystem
  Scope : Scope  NumInputPorts=4
  electric machine filter : Subsystem
  Out1 : Outport
  wires:
  In1/1 -> AxlTrq_to_MtrTrq2/1(In1)
  AxlTrq_to_MtrTrq2/1(MtrTrqCmd) -> Scope/1, electric machine filter/1(trq)  "MtrTrqCmd"
  electric machine filter/1(filtered) -> Scope/2, MotTrqLimit/1  "MtrTrqCmd"
  RegTrqLimit/1(Out1) -> Scope/4, Out1/1  "MtrTrqCmd"
  MotTrqLimit/1 -> Scope/3, RegTrqLimit/1(MotTrqCmd)  "MtrTrqCmd"
  [MotorSpeed] -> RegTrqLimit/2(RPM)
  Mode/1 -> RegTrqLimit/3(mode)

== system Hybrid_P2_Parallel/Controller/HSC/Powertrain Manager/Torque Distribution/IdleMotTrq/AxlTrq_to_MotTrq1 ==
  In1 : Inport
  AxlTrq_to_MtrTrq2 : Subsystem
  MotTrqLimit : Saturate  UpperLimit=350  LowerLimit=-200
  Scope : Scope  NumInputPorts=4
  Subsystem : Subsystem
  electric machine filter : Subsystem
  Out1 : Outport
  wires:
  [MotorSpeed] -> Subsystem/2(RPM)
  MotTrqLimit/1 -> Subsystem/1(In1), Scope/3  "MtrTrqCmd"
  Subsystem/1(Out1) -> Out1/1, Scope/4  "MtrTrqCmd"
  electric machine filter/1(filtered) -> MotTrqLimit/1, Scope/2  "MtrTrqCmd"
  AxlTrq_to_MtrTrq2/1(MtrTrqCmd) -> electric machine filter/1(trq), Scope/1  "MtrTrqCmd"
  In1/1 -> AxlTrq_to_MtrTrq2/1(In1)

== system Hybrid_P2_Parallel/Controller/HSC/Powertrain Manager/Torque Distribution/IdleMotTrq/Idle Torque PID ==
  Setpoint : Inport
  Actual : Inport  Port=2
  Add : Sum  Inputs=+-
  IdleTrqVal : Constant  Value=7
  Kp : Constant  Value=0.2
  Product : Product
  Sum : Sum
  Out1 : Outport
  wires:
  Kp/1 -> Product/2
  Product/1 -> Sum/1
  Setpoint/1 -> Add/1
  Add/1 -> Product/1
  Actual/1 -> Add/2
  Sum/1 -> Out1/1
  IdleTrqVal/1 -> Sum/2

== system Hybrid_P2_Parallel/Controller/HSC/Powertrain Manager/Torque Distribution/Sport Mode Enable/Override Sport Switch ==
  In1 : Inport
  Constant : Constant
  Constant1 : Constant
  Data Type Conversion : DataTypeConversion
  Switch : Switch  Criteria=u2 > Threshold
  Out1 : Outport
  wires:
  In1/1 -> Switch/1
  Switch/1 -> Data Type Conversion/1
  Constant/1 -> Switch/2
  Constant1/1 -> Switch/3
  Data Type Conversion/1 -> Out1/1

== system Hybrid_P2_Parallel/Controller/HSC/Powertrain Manager/Torque Distribution/Supervisory  Control  Logic/VehReady.CS_Mode.Engine_Charge.Drive_Mode.EngTrqCalc/SOC Window Estimation ==
  SOC : Inport
  Constant5 : Constant
  Constant6 : Constant  Value=0
  Memory : Memory  InheritSampleTime=on
  SOC<CS_SOCmin : simulink/Logic and Bit Operations/Compare To Constant  relop=<  const=16  OutDataTypeStr=boolean
  SOC>CS_SOC_min : simulink/Logic and Bit Operations/Compare To Constant  relop=>=  const=19  OutDataTypeStr=boolean
  Switch4 : Switch  Criteria=u2 > Threshold
  Switch5 : Switch  Criteria=u2 > Threshold
  Out1 : Outport
  wires:
  SOC/1 -> SOC<CS_SOCmin/1, SOC>CS_SOC_min/1
  Switch4/1 -> Memory/1, Out1/1
  SOC<CS_SOCmin/1 -> Switch4/2
  SOC>CS_SOC_min/1 -> Switch5/2
  Memory/1 -> Switch5/3
  Constant6/1 -> Switch5/1
  Constant5/1 -> Switch4/1
  Switch5/1 -> Switch4/3

== system Hybrid_P2_Parallel/Controller/HSC/Powertrain Manager/Torque Distribution/Supervisory  Control  Logic/VehReady.CS_Mode.Engine_Charge.Drive_Mode.MotTrqCalc/CS_Switch ==
  note: If CS Switch is not pressed it outputs a zero
      |
      | If CS Switch is pressed:
      | - If the actual SOC < Faked SOC it outputs a 1
      | - If the actual SOC > = (Faked SOC + offset) it outputs a 0
      | - If the  (Faked SOC < SOC < Faked SOC +offset ) it outputs a 0
  SOC : Inport
  Faked_SoC_limit : Inport  Port=2
  CS_On : Inport  Port=3
  Add1 : Sum
  CS_Off : Constant  Value=0
  Constant8 : Constant
  Constant9 : Constant  Value=0
  Memory1 : Memory  InheritSampleTime=on
  Relational Operator : RelationalOperator  Operator=<  OutDataTypeStr=boolean  RndMeth=Nearest
  Relational Operator1 : RelationalOperator  OutDataTypeStr=boolean  RndMeth=Nearest
  SOC_Offset_Cal : Constant  Value=4
  Switch2 : Switch  Criteria=u2 > Threshold
  Switch6 : Switch  Criteria=u2 > Threshold
  Switch7 : Switch  Criteria=u2 > Threshold
  Out1 : Outport
  wires:
  Faked_SoC_limit/1 -> Relational Operator/2, Add1/1
  Switch7/1 -> Switch6/3
  Constant9/1 -> Switch7/1
  Memory1/1 -> Switch7/3
  Relational Operator1/1 -> Switch7/2
  CS_On/1 -> Switch2/2
  SOC/1 -> Relational Operator/1, Relational Operator1/1
  Relational Operator/1 -> Switch6/2
  Constant8/1 -> Switch6/1
  Switch6/1 -> Switch2/1, Memory1/1
  Switch2/1 -> Out1/1
  CS_Off/1 -> Switch2/3
  SOC_Offset_Cal/1 -> Add1/2
  Add1/1 -> Relational Operator1/2
